simulink model "smd"  (R2014b)
settings: Solver=ode45  StartTime=0.0  StopTime=100  RelTol=1e-3
settings Model: Creator=emiller  LastModifiedBy=emiller

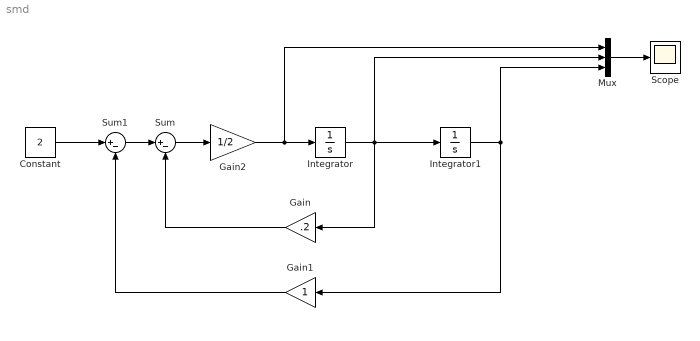
== system smd ==
  Constant : Constant  Value=2
  Gain : Gain  Gain=.2
  Gain1 : Gain
  Gain2 : Gain  Gain=1/2
  Integrator : Integrator
  Integrator1 : Integrator  InitialCondition=5
  Mux : Mux  Inputs=3
  Scope : Scope
  Sum : Sum  Inputs=|+-
  Sum1 : Sum  Inputs=|+-
  wires:
  Integrator/1 -> Mux/2, Gain/1, Integrator1/1
  Integrator1/1 -> Gain1/1, Mux/3
  Mux/1 -> Scope/1
  Gain2/1 -> Mux/1, Integrator/1
  Sum/1 -> Gain2/1
  Gain/1 -> Sum/2
  Gain1/1 -> Sum1/2
  Sum1/1 -> Sum/1
  Constant/1 -> Sum1/1
